simulink model "Decoder2_4"  (R2025b)
settings: Solver=VariableStepAuto  StartTime=0.0  StopTime=10.0  RelTol=1e-3
settings Model: Creator=Johan  LastModifiedBy=Johan

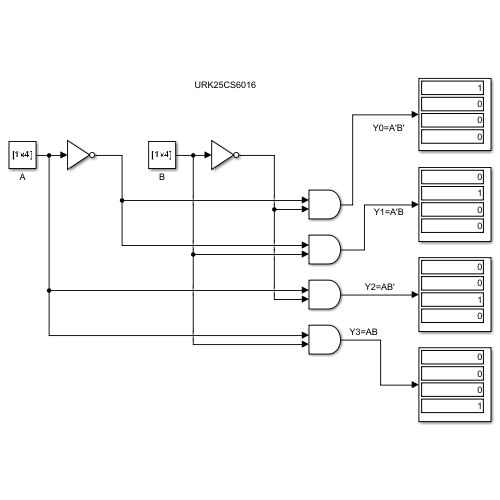
[thumbnail: Simulink's stored preview of the top-level diagram]
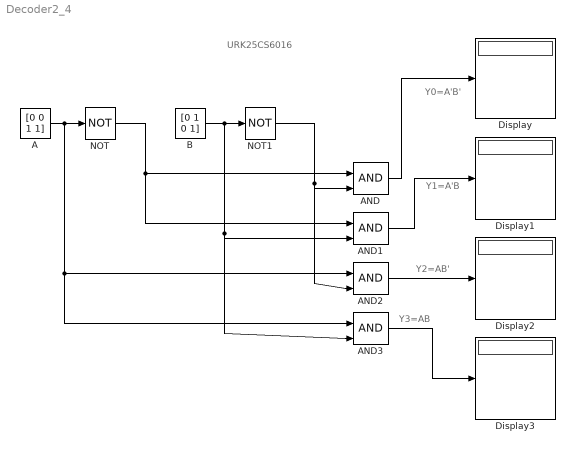
== system Decoder2_4 ==
  note: URK25CS6016
  note: Y0=A'B'
  note: Y1=A'B
  note: Y2=AB'
  note: Y3=AB
  A : Constant  Value=[0 0 1 1]
  AND{,1..3} (4 alike) : Logic  IconShape=distinctive  AllPortsSameDT=off  OutDataTypeStr=boolean
  B : Constant  Value=[0 1 0 1]
  Display{,1..3} (4 alike) : Display
  NOT : Logic  Operator=NOT  IconShape=distinctive  AllPortsSameDT=off  OutDataTypeStr=boolean
  NOT1 : Logic  Operator=NOT  IconShape=distinctive  AllPortsSameDT=off  OutDataTypeStr=boolean
  wires:
  A/1 -> AND2/1, AND3/1, NOT/1
  NOT/1 -> AND1/1, AND/1
  B/1 -> AND3/2, AND1/2, NOT1/1
  NOT1/1 -> AND2/2, AND/2
  AND/1 -> Display/1
  AND1/1 -> Display1/1
  AND2/1 -> Display2/1
  AND3/1 -> Display3/1
